simulink model "system"  (R2023b)
settings: Solver=VariableStepAuto  StartTime=0.0  StopTime=10.0  RelTol=1e-3
model workspace (MAT data in the model file):
  angleqp = Simulink.Parameter
  angleqp.DataType = 'auto'
  angleqp.Complexity = 'real'
  angleqp.Dimensions = [0 0]
  angleqr = Simulink.Parameter
  angleqr.DataType = 'auto'
  angleqr.Complexity = 'real'
  angleqr.Dimensions = [0 0]
  ax = Simulink.Parameter
  ax.DataType = 'auto'
  ax.Complexity = 'real'
  ax.Dimensions = [0 0]
  betar = Simulink.Parameter
  betar.DataType = 'auto'
  betar.Complexity = 'real'
  betar.Dimensions = [0 0]
libraries: slpidlib x1
settings Model: Creator=ritwi  LastModifiedBy=ritwi

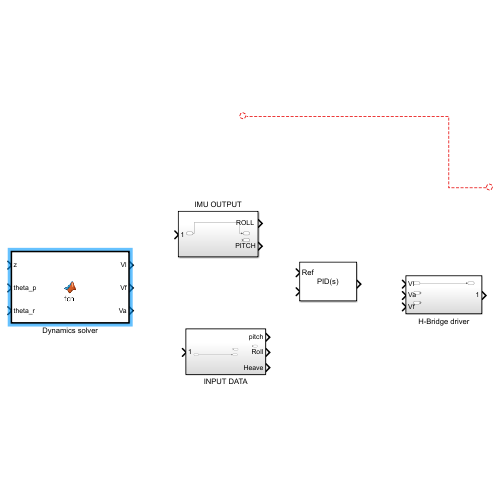
[thumbnail: Simulink's stored preview of the top-level diagram]
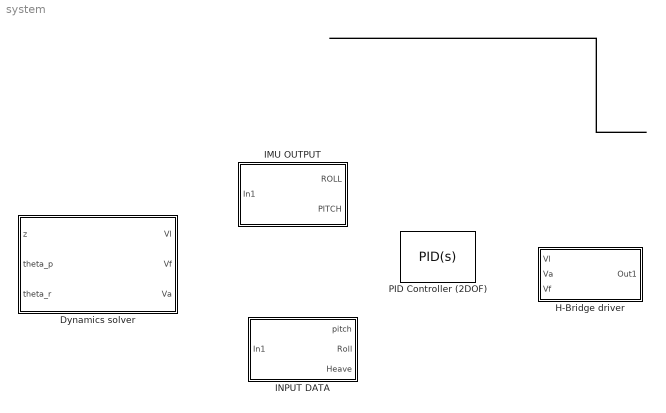
== system system ==
  Dynamics solver : MATLAB Function  TreatAsAtomicUnit=on
  H-Bridge driver : Subsystem
  IMU OUTPUT : Subsystem
  INPUT DATA : Subsystem
  PID Controller (2DOF) : slpidlib/PID Controller (2DOF)  Controller=PID  Form=Parallel  TimeDomain=Continuous-time  UseExternalTs=off  SampleTime=-1  IntegratorMethod=Forward Euler  FilterMethod=Forward Euler  ControllerParametersSource=internal  P=1  I=1  UseKiTs=off  D=0  N=100  UseFilter=on  b=1  c=1  TunerSelectOption=Transfer Function Based (PID Tuner App)  InitialConditionSource=internal  InitialConditionForIntegrator=0  InitialConditionForFilter=0  DifferentiatorICPrevScaledInput=0  ExternalReset=none  TrackingMode=off  Kt=1  LimitOutput=off  SatLimitsSource=internal  UpperSaturationLimit=inf  LowerSaturationLimit=-inf  LinearizeAsGain=on  AntiWindupMode=none  Kb=1  LimitIntegrator=off  UpperIntegratorSaturationLimit=inf  LowerIntegratorSaturationLimit=-inf  POutMin=[]  POutMax=[]  IOutMin=[]  IOutMax=[]  DOutMin=[]  DOutMax=[]  NOutMin=[]  NOutMax=[]  bOutMin=[]  bOutMax=[]  cOutMin=[]  cOutMax=[]  SumOutMin=[]  SumOutMax=[]  SaturationOutMin=[]  SaturationOutMax=[]  PParamMin=[]  PParamMax=[]  IParamMin=[]  IParamMax=[]  DParamMin=[]  DParamMax=[]  NParamMin=[]  NParamMax=[]  bParamMin=[]  bParamMax=[]  cParamMin=[]  cParamMax=[]  KbParamMin=[]  KbParamMax=[]  KtParamMin=[]  KtParamMax=[]  KbOutMin=[]  KbOutMax=[]  KtOutMin=[]  KtOutMax=[]  IntegratorOutMin=[]  IntegratorOutMax=[]  FilterOutMin=[]  FilterOutMax=[]  SumI1OutMin=[]  SumI1OutMax=[]  SumI2OutMin=[]  SumI2OutMax=[]  SumI3OutMin=[]  SumI3OutMax=[]  SumI4OutMin=[]  SumI4OutMax=[]  SumDOutMin=[]  SumDOutMax=[]  Sum1OutMin=[]  Sum1OutMax=[]  Sum2OutMin=[]  Sum2OutMax=[]  Sum3OutMin=[]  Sum3OutMax=[]  DifferentiatorOutMin=[]  DifferentiatorOutMax=[]  FilterDiffOutCoefMin=[]  FilterDiffOutCoefMax=[]  ReciprocalOutMin=[]  ReciprocalOutMax=[]  SumDenOutMin=[]  SumDenOutMax=[]  SumNumOutMin=[]  SumNumOutMax=[]  DivideOutMin=[]  DivideOutMax=[]  UdiffTsProdOutMin=[]  UdiffTsProdOutMax=[]  NTsProdOutMin=[]  NTsProdOutMax=[]  UintegralTsProdOutMin=[]  UintegralTsProdOutMax=[]  UngainTsProdOutMin=[]  UngainTsProdOutMax=[]  ClampingZeroOutDataTypeStr=Inherit: Inherit via back propagation  ClampingZeroOutMin=[]  ClampingZeroOutMax=[]  FilterDenConstantOutDataTypeStr=Inherit: Inherit via back propagation  FilterDenConstantOutMin=[]  FilterDenConstantOutMax=[]  PCopyOutDataTypeStr=Inherit: Inherit via back propagation  PCopyOutMin=[]  PCopyOutMax=[]  NCopyOutDataTypeStr=Inherit: Inherit via back propagation  NCopyOutMin=[]  NCopyOutMax=[]  IntegratorContinuousStateAttributes=''  IntegratorStateMustResolveToSignalObject=off  IntegratorRTWStateStorageClass=Auto  FilterContinuousStateAttributes=''  FilterStateMustResolveToSignalObject=off  FilterRTWStateStorageClass=Auto  ParallelPVariant=InternalParameters  IdealPVariant=Disabled  IVariant=InternalParameters  DVariant=InternalParameters  bVariant=InternalParameters  cVariant=InternalParameters  IntegratorVariant=Continuous  SatVariant=Disabled  AWVariant=Passthrough  PCopyVariant=Disabled  TRVariant=Disabled  FdbkBlocksVariant=Forward  IdealPFdbkVariant=Disabled  SatFdbkVariant=Disabled  DerivativeFilterVariant=ContFilter  NVariant=InternalParameters  NCopyVariant=Disabled  FilterICVariant=InternalICsFilter  IntegratorICVariant=InternalICs  ExternalResetVariant=Disabled  TRSumVariant=Passthrough  SumFdbkVariant=Disabled  SumVariant=Sum_PID  TsampFilterVariant=InternalTs  TsampNgainVariant=Passthrough  TsampIntegralVariant=Disabled_SignalSpec  ExternalSaturationOutDataTypeStr=Inherit: Same as second input
  connections:
  ?

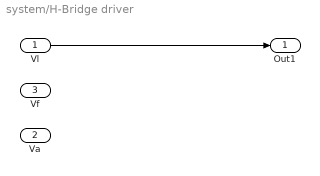
== system system/H-Bridge driver ==
  Vl : Inport
  Va : Inport  Port=2
  Vf : Inport  Port=3
  Out1 : Outport
  wires:
  Vl/1 -> Out1/1

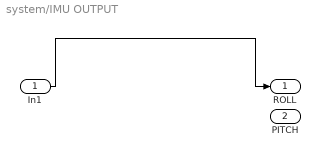
== system system/IMU OUTPUT ==
  In1 : Inport
  "ROLL " : Outport
  PITCH : Outport  Port=2
  wires:
  In1/1 -> "ROLL "/1

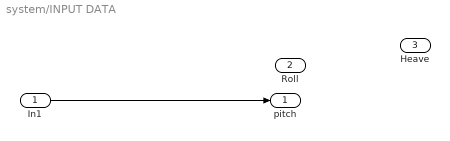
== system system/INPUT DATA ==
  In1 : Inport
  pitch : Outport
  Roll : Outport  Port=2
  Heave : Outport  Port=3
  wires:
  In1/1 -> pitch/1

== matlab function system/Dynamics solver ==
  data: z input; Vl output; theta_p input; theta_r input; Vf output; Va output
function [Vl,Vf,Va]= fcn(z,theta_p,theta_r)

 syms z theta_p theta_r Vl Vf Va beta phi rs
 beta=33.56;
 phi=90-33.56
 rs=200
 eq1=z-Vf+(theta_p*cos(beta)-theta_r*sin(beta))*rs*cos(phi)+(theta_p*sin(beta)+theta_r*cos(beta))*rs*sin(phi);
 eq2=z-Vl-(theta_p*cos(beta)-theta_r*sin(beta))*rs*sin(phi)+(theta_p*sin(beta)+theta_r*cos(beta))*rs*cos(phi);
 eq3=z-Va-(theta_p*cos(beta)-theta_r*sin(beta))*rs*cos(phi)-(theta_p*sin(beta)+theta_r*cos(beta))*rs*sin(phi);

 Vl,Vf,Va=solve(eq1,eq2,eq3,Vl,Vf,Va)
end
